simulink model "velocity_tracking_thresholds"  (R2018b)
settings: Solver=ode8  StartTime=0.0  StopTime=14  FixedStep=0.05  RelTol=1e-3
settings Model: Creator=suvo.ganguli  LastModifiedBy=suvo.ganguli

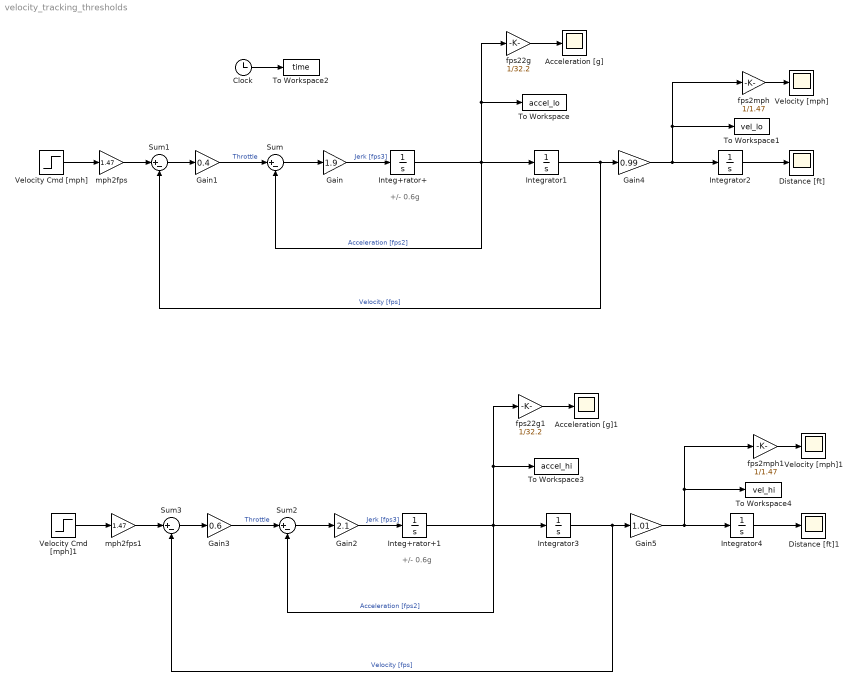
== system velocity_tracking_thresholds ==
  note: +/- 0.6g
  note: +/- 0.6g
  Acceleration [g] : Scope
  Acceleration [g]1 : Scope
  Clock : Clock
  Distance [ft] : Scope
  Distance [ft]1 : Scope
  Gain : Gain  Gain=1.9
  Gain1 : Gain  Gain=0.4
  Gain2 : Gain  Gain=2.1
  Gain3 : Gain  Gain=0.6
  Gain4 : Gain  Gain=0.99
  Gain5 : Gain  Gain=1.01
  Integ+rator+ : Integrator  LimitOutput=on  UpperSaturationLimit=0.6*32.2  LowerSaturationLimit=-0.6*32.2
  Integ+rator+1 : Integrator  LimitOutput=on  UpperSaturationLimit=0.6*32.2  LowerSaturationLimit=-0.6*32.2
  Integrator1 : Integrator  InitialCondition=20*1.47
  Integrator2 : Integrator
  Integrator3 : Integrator  InitialCondition=20*1.47
  Integrator4 : Integrator
  Sum{,1..3} (4 alike) : Sum  Inputs=|+-
  To Workspace : ToWorkspace  VariableName=accel_lo  SampleTime=-1
  To Workspace1 : ToWorkspace  VariableName=vel_lo  SampleTime=-1
  To Workspace2 : ToWorkspace  VariableName=time  SampleTime=-1
  To Workspace3 : ToWorkspace  VariableName=accel_hi  SampleTime=-1
  To Workspace4 : ToWorkspace  VariableName=vel_hi  SampleTime=-1
  Velocity [mph] : Scope
  Velocity [mph]1 : Scope
  Velocity Cmd [mph] : Step  Time=0  Before=20  After=45  SampleTime=0
  Velocity Cmd [mph]1 : Step  Time=0  Before=20  After=45  SampleTime=0
  fps22g : Gain  Gain=1/32.2
  fps22g1 : Gain  Gain=1/32.2
  fps2mph : Gain  Gain=1/1.47
  fps2mph1 : Gain  Gain=1/1.47
  mph2fps : Gain  Gain=1.47
  mph2fps1 : Gain  Gain=1.47
  wires:
  Sum/1 -> Gain/1
  Gain/1 -> Integ+rator+/1  "Jerk [fps3]"
  Integ+rator+/1 -> Integrator1/1, To Workspace/1, fps22g/1, Sum/2  "Acceleration [fps2]"
  Sum1/1 -> Gain1/1
  Integrator1/1 -> Gain4/1, Sum1/2  "Velocity [fps]"
  Gain1/1 -> Sum/1  "Throttle"
  Integrator2/1 -> Distance [ft]/1
  mph2fps/1 -> Sum1/1
  fps2mph/1 -> Velocity [mph]/1
  fps22g/1 -> Acceleration [g]/1
  Velocity Cmd [mph]/1 -> mph2fps/1
  Clock/1 -> To Workspace2/1
  Gain4/1 -> Integrator2/1, To Workspace1/1, fps2mph/1
  Gain3/1 -> Sum2/1  "Throttle"
  Velocity Cmd [mph]1/1 -> mph2fps1/1
  fps2mph1/1 -> Velocity [mph]1/1
  fps22g1/1 -> Acceleration [g]1/1
  Integrator4/1 -> Distance [ft]1/1
  Sum3/1 -> Gain3/1
  Sum2/1 -> Gain2/1
  Integrator3/1 -> Gain5/1, Sum3/2  "Velocity [fps]"
  Gain5/1 -> Integrator4/1, To Workspace4/1, fps2mph1/1
  mph2fps1/1 -> Sum3/1
  Integ+rator+1/1 -> Integrator3/1, To Workspace3/1, fps22g1/1, Sum2/2  "Acceleration [fps2]"
  Gain2/1 -> Integ+rator+1/1  "Jerk [fps3]"
